simulink model "TwoBitMUX"  (R2017b)
settings: Solver=VariableStepAuto  StartTime=0.0  StopTime=10.0  RelTol=1e-3
libraries: hdlsllib x21
settings Model: Creator=Ray  LastModifiedBy=Ray

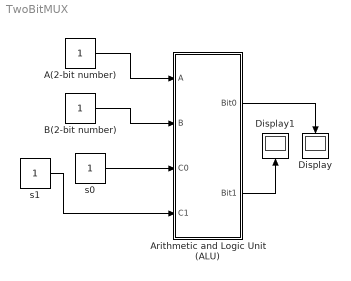
== system TwoBitMUX ==
  A(2-bit number) : Constant  OutDataTypeStr=uint8  SampleTime=1
  Arithmetic and Logic Unit (ALU) : Subsystem  TreatAsAtomicUnit=on
  B(2-bit number) : Constant  OutDataTypeStr=uint8  SampleTime=1
  Display : Display
  Display1 : Display
  s0 : Constant  OutDataTypeStr=boolean  SampleTime=1
  s1 : Constant  OutDataTypeStr=boolean  SampleTime=1
  wires:
  Arithmetic and Logic Unit (ALU)/1(Bit0) -> Display/1
  A(2-bit number)/1 -> Arithmetic and Logic Unit (ALU)/1(A)
  B(2-bit number)/1 -> Arithmetic and Logic Unit (ALU)/2(B)
  s0/1 -> Arithmetic and Logic Unit (ALU)/3(C0)
  s1/1 -> Arithmetic and Logic Unit (ALU)/4(C1)
  Arithmetic and Logic Unit (ALU)/2(Bit1) -> Display1/1

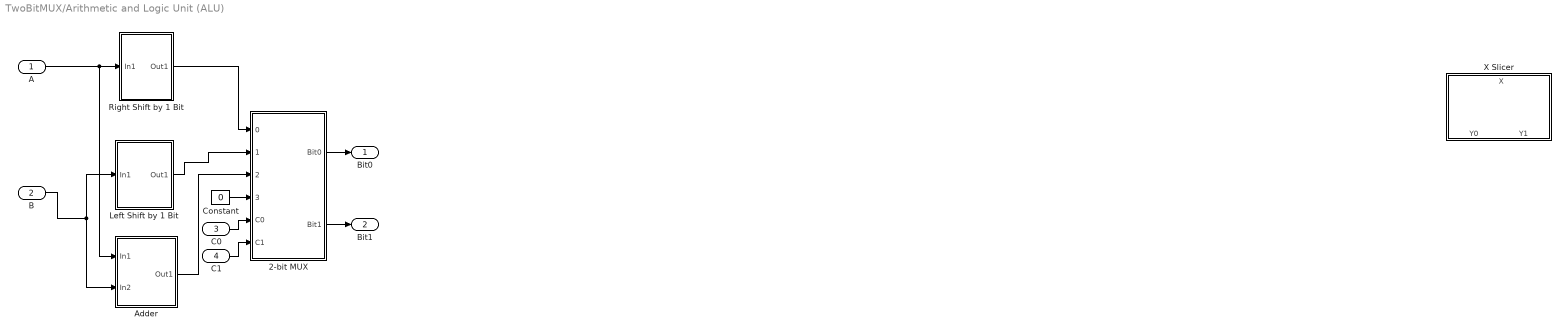
== system TwoBitMUX/Arithmetic and Logic Unit (ALU) ==
  A : Inport  OutDataTypeStr=uint8  SampleTime=1
  B : Inport  Port=2  OutDataTypeStr=uint8  SampleTime=1
  C0 : Inport  Port=3  OutDataTypeStr=boolean  SampleTime=1
  C1 : Inport  Port=4  OutDataTypeStr=boolean  SampleTime=1
  2-bit MUX : Subsystem
  Adder : Subsystem
  Constant : Constant  Value=0  OutDataTypeStr=uint8  SampleTime=1
  Left Shift by 1 Bit : Subsystem
  Right Shift by 1 Bit : Subsystem
  X Slicer : Subsystem
  Bit0 : Outport
  Bit1 : Outport  Port=2
  wires:
  Adder/1(Out1) -> 2-bit MUX/3(2)
  B/1 -> Adder/2(In2), Left Shift by 1 Bit/1(In1)
  A/1 -> Right Shift by 1 Bit/1(In1), Adder/1(In1)
  C0/1 -> 2-bit MUX/5(C0)
  C1/1 -> 2-bit MUX/6(C1)
  Constant/1 -> 2-bit MUX/4(3)
  2-bit MUX/1(Bit0) -> Bit0/1
  2-bit MUX/2(Bit1) -> Bit1/1
  Left Shift by 1 Bit/1(Out1) -> 2-bit MUX/2(1)
  Right Shift by 1 Bit/1(Out1) -> 2-bit MUX/1(0)

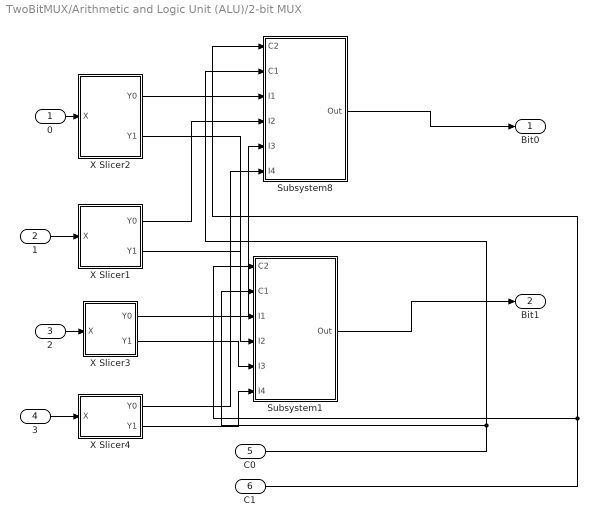
== system TwoBitMUX/Arithmetic and Logic Unit (ALU)/2-bit MUX ==
  0 : Inport  OutDataTypeStr=uint8  SampleTime=1
  1 : Inport  Port=2  OutDataTypeStr=uint8  SampleTime=1
  2 : Inport  Port=3  OutDataTypeStr=uint8  SampleTime=1
  3 : Inport  Port=4  OutDataTypeStr=uint8  SampleTime=1
  C0 : Inport  Port=5  OutDataTypeStr=boolean  SampleTime=1
  C1 : Inport  Port=6  OutDataTypeStr=boolean  SampleTime=1
  Subsystem1 : Subsystem
  Subsystem8 : Subsystem
  X Slicer1 : Subsystem
  X Slicer2 : Subsystem
  X Slicer3 : Subsystem
  X Slicer4 : Subsystem
  Bit0 : Outport  OutDataTypeStr=boolean  SampleTime=1
  Bit1 : Outport  Port=2  OutDataTypeStr=boolean  SampleTime=1
  wires:
  1/1 -> X Slicer1/1(X)
  X Slicer3/2(Y1) -> Subsystem1/5(I3)
  X Slicer1/1(Y0) -> Subsystem8/4(I2)
  X Slicer1/2(Y1) -> Subsystem1/4(I2)
  C1/1 -> Subsystem8/1(C2), Subsystem1/1(C2)
  X Slicer2/2(Y1) -> Subsystem1/3(I1)
  C0/1 -> Subsystem8/2(C1), Subsystem1/2(C1)
  X Slicer4/1(Y0) -> Subsystem8/6(I4)
  0/1 -> X Slicer2/1(X)
  X Slicer3/1(Y0) -> Subsystem8/5(I3)
  X Slicer4/2(Y1) -> Subsystem1/6(I4)
  X Slicer2/1(Y0) -> Subsystem8/3(I1)
  2/1 -> X Slicer3/1(X)
  3/1 -> X Slicer4/1(X)
  Subsystem8/1(Out) -> Bit0/1
  Subsystem1/1(Out) -> Bit1/1

== system TwoBitMUX/Arithmetic and Logic Unit (ALU)/Adder ==
  In1 : Inport
  In2 : Inport  Port=2
  8-bit Adder : Subsystem
  Bit Concat : Subsystem
  X Slicer : Subsystem
  X Slicer1 : Subsystem
  Out1 : Outport
  wires:
  Bit Concat/1(Out1) -> Out1/1
  In1/1 -> X Slicer/1(X)
  In2/1 -> X Slicer1/1(X)
  8-bit Adder/8(Out8) -> Bit Concat/1(In1)
  8-bit Adder/7(Out7) -> Bit Concat/2(In2)
  8-bit Adder/6(Out6) -> Bit Concat/3(In3)
  8-bit Adder/5(Out5) -> Bit Concat/4(In4)
  8-bit Adder/4(Out4) -> Bit Concat/5(In5)
  8-bit Adder/3(Out3) -> Bit Concat/6(In6)
  8-bit Adder/2(Out2) -> Bit Concat/7(In7)
  8-bit Adder/1(Out1) -> Bit Concat/8(In8)
  X Slicer/1(Y0) -> 8-bit Adder/1(A1)
  X Slicer/2(Y1) -> 8-bit Adder/3(A2)
  X Slicer1/1(Y0) -> 8-bit Adder/2(B1)
  X Slicer1/2(Y1) -> 8-bit Adder/10(B2)

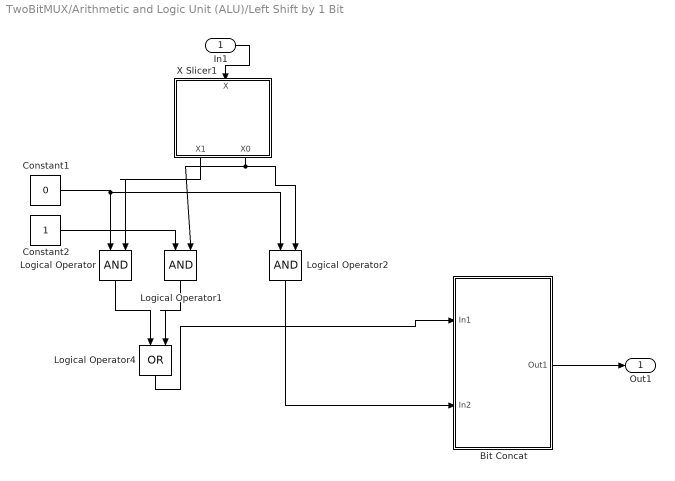
== system TwoBitMUX/Arithmetic and Logic Unit (ALU)/Left Shift by 1 Bit ==
  In1 : Inport
  Bit Concat : Subsystem
  Constant1 : Constant  Value=0  OutDataTypeStr=boolean  SampleTime=1
  Constant2 : Constant  OutDataTypeStr=boolean  SampleTime=1
  Logical Operator : Logic  IconShape=distinctive  AllPortsSameDT=off  OutDataTypeStr=boolean
  Logical Operator1 : Logic  IconShape=distinctive  AllPortsSameDT=off  OutDataTypeStr=boolean
  Logical Operator2 : Logic  IconShape=distinctive  AllPortsSameDT=off  OutDataTypeStr=boolean
  Logical Operator4 : Logic  Operator=OR  IconShape=distinctive  AllPortsSameDT=off  OutDataTypeStr=boolean
  X Slicer1 : Subsystem
  Out1 : Outport
  wires:
  Logical Operator4/1 -> Bit Concat/1(In1)
  X Slicer1/1(X1) -> Logical Operator/2
  Logical Operator2/1 -> Bit Concat/2(In2)
  Constant1/1 -> Logical Operator2/1, Logical Operator/1
  Logical Operator1/1 -> Logical Operator4/2
  X Slicer1/2(X0) -> Logical Operator2/2, Logical Operator1/2
  In1/1 -> X Slicer1/1(X)
  Constant2/1 -> Logical Operator1/1
  Logical Operator/1 -> Logical Operator4/1
  Bit Concat/1(Out1) -> Out1/1

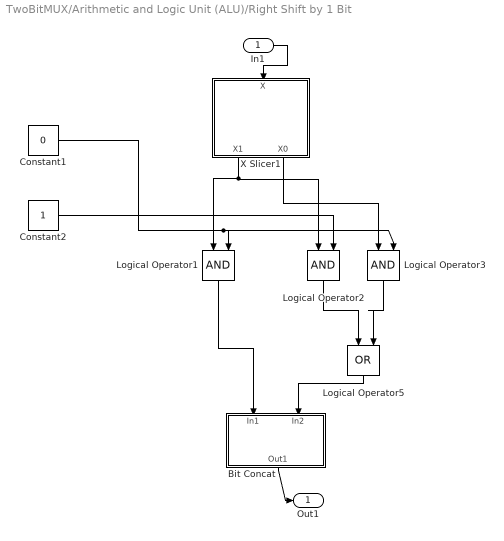
== system TwoBitMUX/Arithmetic and Logic Unit (ALU)/Right Shift by 1 Bit ==
  In1 : Inport
  Bit Concat : Subsystem
  Constant1 : Constant  Value=0  OutDataTypeStr=boolean  SampleTime=1
  Constant2 : Constant  OutDataTypeStr=boolean  SampleTime=1
  Logical Operator1 : Logic  IconShape=distinctive  AllPortsSameDT=off  OutDataTypeStr=boolean
  Logical Operator2 : Logic  IconShape=distinctive  AllPortsSameDT=off  OutDataTypeStr=boolean
  Logical Operator3 : Logic  IconShape=distinctive  AllPortsSameDT=off  OutDataTypeStr=boolean
  Logical Operator5 : Logic  Operator=OR  IconShape=distinctive  AllPortsSameDT=off  OutDataTypeStr=boolean
  X Slicer1 : Subsystem
  Out1 : Outport
  wires:
  In1/1 -> X Slicer1/1(X)
  Logical Operator5/1 -> Bit Concat/2(In2)
  Bit Concat/1(Out1) -> Out1/1
  X Slicer1/2(X0) -> Logical Operator3/1
  X Slicer1/1(X1) -> Logical Operator1/1, Logical Operator2/1
  Constant1/1 -> Logical Operator1/2, Logical Operator3/2
  Constant2/1 -> Logical Operator2/2
  Logical Operator1/1 -> Bit Concat/1(In1)
  Logical Operator3/1 -> Logical Operator5/2
  Logical Operator2/1 -> Logical Operator5/1

== system TwoBitMUX/Arithmetic and Logic Unit (ALU)/X Slicer ==
  X : Inport  OutDataTypeStr=uint8  SampleTime=1
  Bit Slice6 : hdlsllib/Logic and Bit Operations/Bit Slice  lidx=1  ridx=1
  Bit Slice7 : hdlsllib/Logic and Bit Operations/Bit Slice  lidx=0  ridx=0
  Data Type Conversion6 : DataTypeConversion  OutDataTypeStr=boolean
  Data Type Conversion7 : DataTypeConversion  OutDataTypeStr=boolean
  Y0 : Outport
  Y1 : Outport  Port=2
  wires:
  X/1 -> Bit Slice6/1, Bit Slice7/1
  Data Type Conversion6/1 -> Y1/1
  Bit Slice6/1 -> Data Type Conversion6/1
  Data Type Conversion7/1 -> Y0/1
  Bit Slice7/1 -> Data Type Conversion7/1

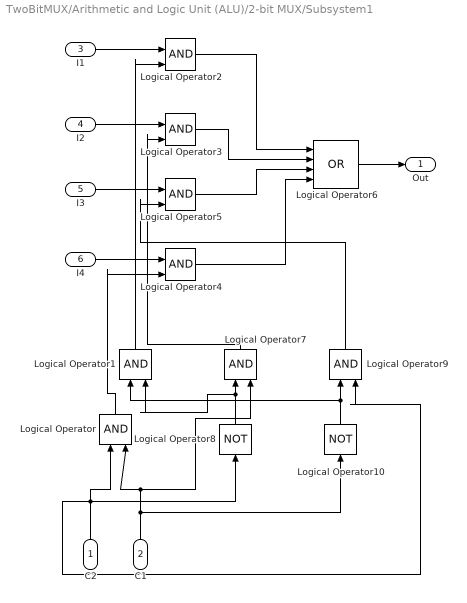
== system TwoBitMUX/Arithmetic and Logic Unit (ALU)/2-bit MUX/Subsystem1 ==
  C2 : Inport
  C1 : Inport  Port=2
  I1 : Inport  Port=3
  I2 : Inport  Port=4
  I3 : Inport  Port=5
  I4 : Inport  Port=6
  Logical Operator{,1..5,7,9} (8 alike) : Logic  IconShape=distinctive  AllPortsSameDT=off  OutDataTypeStr=boolean
  Logical Operator10 : Logic  Operator=NOT  IconShape=distinctive  AllPortsSameDT=off  OutDataTypeStr=boolean
  Logical Operator6 : Logic  Operator=OR  Inputs=4  IconShape=distinctive  AllPortsSameDT=off  OutDataTypeStr=boolean
  Logical Operator8 : Logic  Operator=NOT  IconShape=distinctive  AllPortsSameDT=off  OutDataTypeStr=boolean
  Out : Outport
  wires:
  I1/1 -> Logical Operator2/1
  I3/1 -> Logical Operator5/1
  Logical Operator4/1 -> Logical Operator6/4
  Logical Operator3/1 -> Logical Operator6/2
  C1/1 -> Logical Operator10/1, Logical Operator/2, Logical Operator7/2
  C2/1 -> Logical Operator9/2, Logical Operator/1, Logical Operator8/1
  Logical Operator10/1 -> Logical Operator1/1, Logical Operator9/1
  Logical Operator/1 -> Logical Operator4/2
  Logical Operator7/1 -> Logical Operator3/2
  I2/1 -> Logical Operator3/1
  Logical Operator2/1 -> Logical Operator6/1
  Logical Operator9/1 -> Logical Operator5/2
  I4/1 -> Logical Operator4/1
  Logical Operator5/1 -> Logical Operator6/3
  Logical Operator6/1 -> Out/1
  Logical Operator8/1 -> Logical Operator1/2, Logical Operator7/1
  Logical Operator1/1 -> Logical Operator2/2

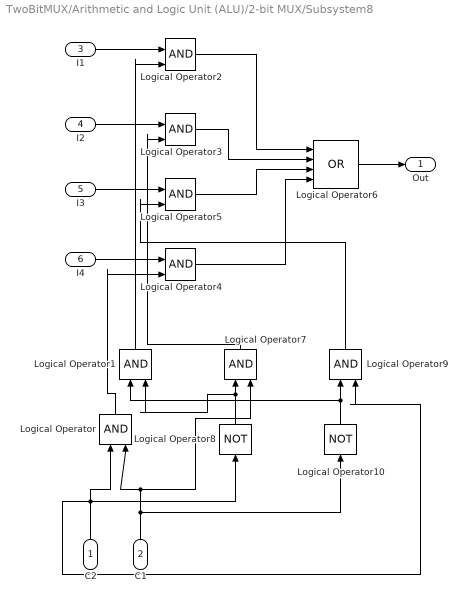
== system TwoBitMUX/Arithmetic and Logic Unit (ALU)/2-bit MUX/Subsystem8 ==
  C2 : Inport
  C1 : Inport  Port=2
  I1 : Inport  Port=3
  I2 : Inport  Port=4
  I3 : Inport  Port=5
  I4 : Inport  Port=6
  Logical Operator{,1..5,7,9} (8 alike) : Logic  IconShape=distinctive  AllPortsSameDT=off  OutDataTypeStr=boolean
  Logical Operator10 : Logic  Operator=NOT  IconShape=distinctive  AllPortsSameDT=off  OutDataTypeStr=boolean
  Logical Operator6 : Logic  Operator=OR  Inputs=4  IconShape=distinctive  AllPortsSameDT=off  OutDataTypeStr=boolean
  Logical Operator8 : Logic  Operator=NOT  IconShape=distinctive  AllPortsSameDT=off  OutDataTypeStr=boolean
  Out : Outport
  wires:
  I1/1 -> Logical Operator2/1
  I3/1 -> Logical Operator5/1
  Logical Operator4/1 -> Logical Operator6/4
  Logical Operator3/1 -> Logical Operator6/2
  C1/1 -> Logical Operator10/1, Logical Operator/2, Logical Operator7/2
  C2/1 -> Logical Operator9/2, Logical Operator/1, Logical Operator8/1
  Logical Operator10/1 -> Logical Operator1/1, Logical Operator9/1
  Logical Operator/1 -> Logical Operator4/2
  Logical Operator7/1 -> Logical Operator3/2
  I2/1 -> Logical Operator3/1
  Logical Operator2/1 -> Logical Operator6/1
  Logical Operator9/1 -> Logical Operator5/2
  I4/1 -> Logical Operator4/1
  Logical Operator5/1 -> Logical Operator6/3
  Logical Operator6/1 -> Out/1
  Logical Operator8/1 -> Logical Operator1/2, Logical Operator7/1
  Logical Operator1/1 -> Logical Operator2/2

== system TwoBitMUX/Arithmetic and Logic Unit (ALU)/2-bit MUX/X Slicer1 ==
  X : Inport  OutDataTypeStr=uint8  SampleTime=1
  Bit Slice6 : hdlsllib/Logic and Bit Operations/Bit Slice  lidx=1  ridx=1
  Bit Slice7 : hdlsllib/Logic and Bit Operations/Bit Slice  lidx=0  ridx=0
  Data Type Conversion6 : DataTypeConversion  OutDataTypeStr=boolean
  Data Type Conversion7 : DataTypeConversion  OutDataTypeStr=boolean
  Y0 : Outport  OutDataTypeStr=boolean  SampleTime=1
  Y1 : Outport  Port=2  OutDataTypeStr=boolean  SampleTime=1
  wires:
  X/1 -> Bit Slice6/1, Bit Slice7/1
  Data Type Conversion6/1 -> Y1/1
  Bit Slice6/1 -> Data Type Conversion6/1
  Data Type Conversion7/1 -> Y0/1
  Bit Slice7/1 -> Data Type Conversion7/1

== system TwoBitMUX/Arithmetic and Logic Unit (ALU)/2-bit MUX/X Slicer2 ==
  X : Inport  OutDataTypeStr=uint8  SampleTime=1
  Bit Slice6 : hdlsllib/Logic and Bit Operations/Bit Slice  lidx=1  ridx=1
  Bit Slice7 : hdlsllib/Logic and Bit Operations/Bit Slice  lidx=0  ridx=0
  Data Type Conversion6 : DataTypeConversion  OutDataTypeStr=boolean
  Data Type Conversion7 : DataTypeConversion  OutDataTypeStr=boolean
  Y0 : Outport  OutDataTypeStr=boolean  SampleTime=1
  Y1 : Outport  Port=2  OutDataTypeStr=boolean  SampleTime=1
  wires:
  X/1 -> Bit Slice6/1, Bit Slice7/1
  Data Type Conversion6/1 -> Y1/1
  Bit Slice6/1 -> Data Type Conversion6/1
  Data Type Conversion7/1 -> Y0/1
  Bit Slice7/1 -> Data Type Conversion7/1

== system TwoBitMUX/Arithmetic and Logic Unit (ALU)/2-bit MUX/X Slicer3 ==
  X : Inport  OutDataTypeStr=uint8  SampleTime=1
  Bit Slice6 : hdlsllib/Logic and Bit Operations/Bit Slice  lidx=1  ridx=1
  Bit Slice7 : hdlsllib/Logic and Bit Operations/Bit Slice  lidx=0  ridx=0
  Data Type Conversion6 : DataTypeConversion  OutDataTypeStr=boolean
  Data Type Conversion7 : DataTypeConversion  OutDataTypeStr=boolean
  Y0 : Outport  OutDataTypeStr=boolean  SampleTime=1
  Y1 : Outport  Port=2  OutDataTypeStr=boolean  SampleTime=1
  wires:
  X/1 -> Bit Slice6/1, Bit Slice7/1
  Data Type Conversion6/1 -> Y1/1
  Bit Slice6/1 -> Data Type Conversion6/1
  Data Type Conversion7/1 -> Y0/1
  Bit Slice7/1 -> Data Type Conversion7/1

== system TwoBitMUX/Arithmetic and Logic Unit (ALU)/2-bit MUX/X Slicer4 ==
  X : Inport  OutDataTypeStr=uint8  SampleTime=1
  Bit Slice6 : hdlsllib/Logic and Bit Operations/Bit Slice  lidx=1  ridx=1
  Bit Slice7 : hdlsllib/Logic and Bit Operations/Bit Slice  lidx=0  ridx=0
  Data Type Conversion6 : DataTypeConversion  OutDataTypeStr=boolean
  Data Type Conversion7 : DataTypeConversion  OutDataTypeStr=boolean
  Y0 : Outport  OutDataTypeStr=boolean  SampleTime=1
  Y1 : Outport  Port=2  OutDataTypeStr=boolean  SampleTime=1
  wires:
  X/1 -> Bit Slice6/1, Bit Slice7/1
  Data Type Conversion6/1 -> Y1/1
  Bit Slice6/1 -> Data Type Conversion6/1
  Data Type Conversion7/1 -> Y0/1
  Bit Slice7/1 -> Data Type Conversion7/1

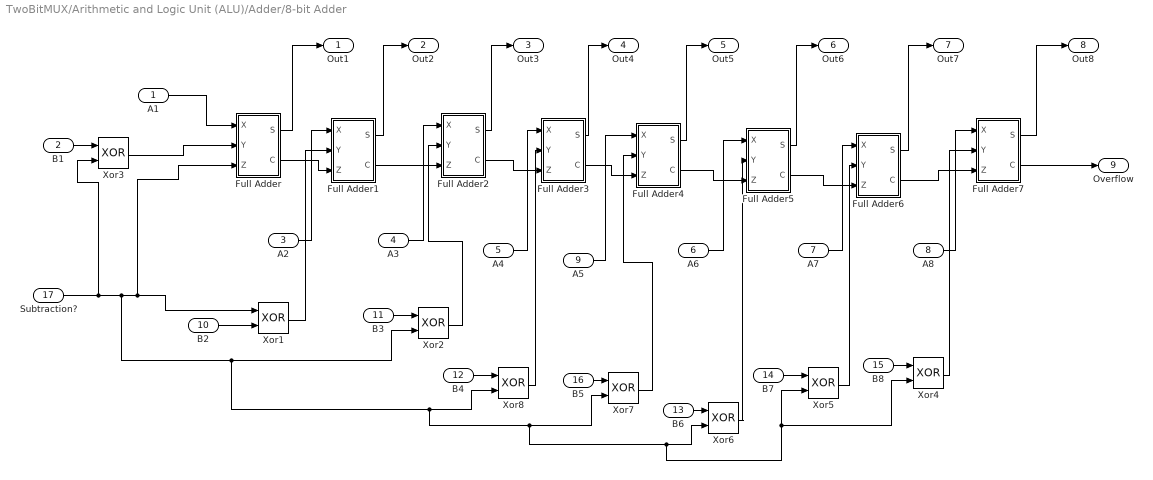
== system TwoBitMUX/Arithmetic and Logic Unit (ALU)/Adder/8-bit Adder ==
  A1 : Inport
  B1 : Inport  Port=2
  A2 : Inport  Port=3
  A3 : Inport  Port=4
  A4 : Inport  Port=5
  A6 : Inport  Port=6
  A7 : Inport  Port=7
  A8 : Inport  Port=8
  A5 : Inport  Port=9
  B2 : Inport  Port=10
  B3 : Inport  Port=11
  B4 : Inport  Port=12
  B6 : Inport  Port=13
  B7 : Inport  Port=14
  B8 : Inport  Port=15
  B5 : Inport  Port=16
  Subtraction? : Inport  Port=17  OutDataTypeStr=boolean
  Full Adder : Subsystem
  Full Adder1 : Subsystem
  Full Adder2 : Subsystem
  Full Adder3 : Subsystem
  Full Adder4 : Subsystem
  Full Adder5 : Subsystem
  Full Adder6 : Subsystem
  Full Adder7 : Subsystem
  Xor{1..8} (8 alike) : Logic  Operator=XOR  AllPortsSameDT=off  OutDataTypeStr=boolean
  Out1 : Outport  OutDataTypeStr=boolean
  Out2 : Outport  Port=2  OutDataTypeStr=boolean
  Out3 : Outport  Port=3  OutDataTypeStr=boolean
  Out4 : Outport  Port=4  OutDataTypeStr=boolean
  Out5 : Outport  Port=5  OutDataTypeStr=boolean
  Out6 : Outport  Port=6  OutDataTypeStr=boolean
  Out7 : Outport  Port=7  OutDataTypeStr=boolean
  Out8 : Outport  Port=8  OutDataTypeStr=boolean
  Overflow : Outport  Port=9  OutDataTypeStr=boolean
  wires:
  Full Adder7/2(C) -> Overflow/1
  Full Adder5/2(C) -> Full Adder6/3(Z)
  Full Adder7/1(S) -> Out8/1
  Full Adder4/2(C) -> Full Adder5/3(Z)
  Full Adder/2(C) -> Full Adder1/3(Z)
  Full Adder6/2(C) -> Full Adder7/3(Z)
  Full Adder6/1(S) -> Out7/1
  Full Adder2/2(C) -> Full Adder3/3(Z)
  Full Adder4/1(S) -> Out5/1
  A2/1 -> Full Adder1/1(X)
  A5/1 -> Full Adder4/1(X)
  Full Adder1/1(S) -> Out2/1
  A7/1 -> Full Adder6/1(X)
  Full Adder5/1(S) -> Out6/1
  A1/1 -> Full Adder/1(X)
  A8/1 -> Full Adder7/1(X)
  A6/1 -> Full Adder5/1(X)
  A4/1 -> Full Adder3/1(X)
  Full Adder3/1(S) -> Out4/1
  Full Adder/1(S) -> Out1/1
  Full Adder1/2(C) -> Full Adder2/3(Z)
  A3/1 -> Full Adder2/1(X)
  Full Adder3/2(C) -> Full Adder4/3(Z)
  Full Adder2/1(S) -> Out3/1
  B2/1 -> Xor1/2
  Subtraction?/1 -> Xor3/2, Xor4/2, Xor5/2, Xor6/2, Xor7/2, Xor8/2, Xor2/2, Full Adder/3(Z), Xor1/1
  Xor1/1 -> Full Adder1/2(Y)
  Xor2/1 -> Full Adder2/2(Y)
  B3/1 -> Xor2/1
  B4/1 -> Xor8/1
  Xor8/1 -> Full Adder3/2(Y)
  B5/1 -> Xor7/1
  Xor7/1 -> Full Adder4/2(Y)
  B6/1 -> Xor6/1
  Xor6/1 -> Full Adder5/2(Y)
  B7/1 -> Xor5/1
  Xor5/1 -> Full Adder6/2(Y)
  Xor4/1 -> Full Adder7/2(Y)
  B8/1 -> Xor4/1
  Xor3/1 -> Full Adder/2(Y)
  B1/1 -> Xor3/1

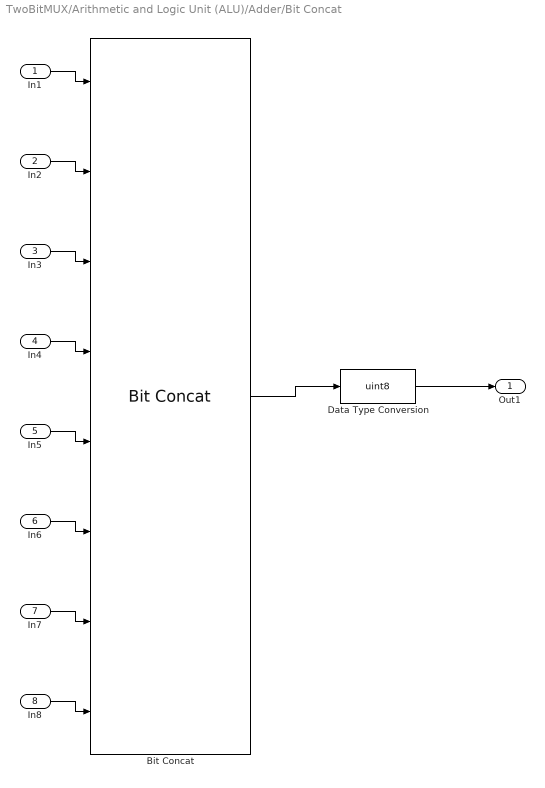
== system TwoBitMUX/Arithmetic and Logic Unit (ALU)/Adder/Bit Concat ==
  In1 : Inport
  In2 : Inport  Port=2
  In3 : Inport  Port=3
  In4 : Inport  Port=4
  In5 : Inport  Port=5
  In6 : Inport  Port=6
  In7 : Inport  Port=7
  In8 : Inport  Port=8
  Bit Concat : hdlsllib/Logic and Bit Operations/Bit Concat  numInputs=8
      settings: SourceProductName=HDL Coder  SourceProductBaseCode=HD
  Data Type Conversion : DataTypeConversion  OutDataTypeStr=uint8
  Out1 : Outport
  wires:
  Data Type Conversion/1 -> Out1/1
  In1/1 -> Bit Concat/1
  In4/1 -> Bit Concat/4
  In2/1 -> Bit Concat/2
  In3/1 -> Bit Concat/3
  In5/1 -> Bit Concat/5
  In6/1 -> Bit Concat/6
  In7/1 -> Bit Concat/7
  In8/1 -> Bit Concat/8
  Bit Concat/1 -> Data Type Conversion/1

== system TwoBitMUX/Arithmetic and Logic Unit (ALU)/Adder/X Slicer ==
  X : Inport  OutDataTypeStr=uint8  SampleTime=1
  Bit Slice6 : hdlsllib/Logic and Bit Operations/Bit Slice  lidx=1  ridx=1
  Bit Slice7 : hdlsllib/Logic and Bit Operations/Bit Slice  lidx=0  ridx=0
  Data Type Conversion6 : DataTypeConversion  OutDataTypeStr=boolean
  Data Type Conversion7 : DataTypeConversion  OutDataTypeStr=boolean
  Y0 : Outport
  Y1 : Outport  Port=2
  wires:
  X/1 -> Bit Slice6/1, Bit Slice7/1
  Data Type Conversion6/1 -> Y1/1
  Bit Slice6/1 -> Data Type Conversion6/1
  Data Type Conversion7/1 -> Y0/1
  Bit Slice7/1 -> Data Type Conversion7/1

== system TwoBitMUX/Arithmetic and Logic Unit (ALU)/Adder/X Slicer1 ==
  X : Inport  OutDataTypeStr=uint8  SampleTime=1
  Bit Slice6 : hdlsllib/Logic and Bit Operations/Bit Slice  lidx=1  ridx=1
  Bit Slice7 : hdlsllib/Logic and Bit Operations/Bit Slice  lidx=0  ridx=0
  Data Type Conversion6 : DataTypeConversion  OutDataTypeStr=boolean
  Data Type Conversion7 : DataTypeConversion  OutDataTypeStr=boolean
  Y0 : Outport
  Y1 : Outport  Port=2
  wires:
  X/1 -> Bit Slice6/1, Bit Slice7/1
  Data Type Conversion6/1 -> Y1/1
  Bit Slice6/1 -> Data Type Conversion6/1
  Data Type Conversion7/1 -> Y0/1
  Bit Slice7/1 -> Data Type Conversion7/1

== system TwoBitMUX/Arithmetic and Logic Unit (ALU)/Left Shift by 1 Bit/Bit Concat ==
  In1 : Inport
  In2 : Inport  Port=2
  Bit Concat : hdlsllib/Logic and Bit Operations/Bit Concat  numInputs=2
      settings: SourceProductName=HDL Coder  SourceProductBaseCode=HD
  Data Type Conversion : DataTypeConversion  OutDataTypeStr=uint8
  Out1 : Outport
  wires:
  Data Type Conversion/1 -> Out1/1
  Bit Concat/1 -> Data Type Conversion/1
  In2/1 -> Bit Concat/2
  In1/1 -> Bit Concat/1

== system TwoBitMUX/Arithmetic and Logic Unit (ALU)/Left Shift by 1 Bit/X Slicer1 ==
  X : Inport  OutDataTypeStr=uint8  SampleTime=1
  Bit Slice6 : hdlsllib/Logic and Bit Operations/Bit Slice  lidx=1  ridx=1
  Bit Slice7 : hdlsllib/Logic and Bit Operations/Bit Slice  lidx=0  ridx=0
  Data Type Conversion6 : DataTypeConversion  OutDataTypeStr=boolean
  Data Type Conversion7 : DataTypeConversion  OutDataTypeStr=boolean
  X1 : Outport
  X0 : Outport  Port=2
  wires:
  X/1 -> Bit Slice6/1, Bit Slice7/1
  Data Type Conversion6/1 -> X1/1
  Bit Slice6/1 -> Data Type Conversion6/1
  Data Type Conversion7/1 -> X0/1
  Bit Slice7/1 -> Data Type Conversion7/1

== system TwoBitMUX/Arithmetic and Logic Unit (ALU)/Right Shift by 1 Bit/Bit Concat ==
  In1 : Inport
  In2 : Inport  Port=2
  Bit Concat : hdlsllib/Logic and Bit Operations/Bit Concat  numInputs=2
      settings: SourceProductName=HDL Coder  SourceProductBaseCode=HD
  Data Type Conversion : DataTypeConversion  OutDataTypeStr=uint8
  Out1 : Outport
  wires:
  Data Type Conversion/1 -> Out1/1
  Bit Concat/1 -> Data Type Conversion/1
  In2/1 -> Bit Concat/2
  In1/1 -> Bit Concat/1

== system TwoBitMUX/Arithmetic and Logic Unit (ALU)/Right Shift by 1 Bit/X Slicer1 ==
  X : Inport  OutDataTypeStr=uint8  SampleTime=1
  Bit Slice6 : hdlsllib/Logic and Bit Operations/Bit Slice  lidx=1  ridx=1
  Bit Slice7 : hdlsllib/Logic and Bit Operations/Bit Slice  lidx=0  ridx=0
  Data Type Conversion6 : DataTypeConversion  OutDataTypeStr=boolean
  Data Type Conversion7 : DataTypeConversion  OutDataTypeStr=boolean
  X1 : Outport
  X0 : Outport  Port=2
  wires:
  X/1 -> Bit Slice6/1, Bit Slice7/1
  Data Type Conversion6/1 -> X1/1
  Bit Slice6/1 -> Data Type Conversion6/1
  Data Type Conversion7/1 -> X0/1
  Bit Slice7/1 -> Data Type Conversion7/1

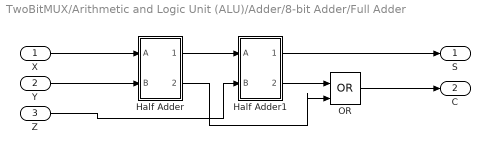
== system TwoBitMUX/Arithmetic and Logic Unit (ALU)/Adder/8-bit Adder/Full Adder ==
  X : Inport
  Y : Inport  Port=2
  Z : Inport  Port=3
  Half Adder : Subsystem
  Half Adder1 : Subsystem
  OR : Logic  Operator=OR  IconShape=distinctive  AllPortsSameDT=off  OutDataTypeStr=boolean
  S : Outport
  C : Outport  Port=2
  wires:
  Half Adder1/1(Sum) -> S/1
  Half Adder/1(Sum) -> Half Adder1/1(A)
  Half Adder/2(Carry) -> OR/2
  X/1 -> Half Adder/1(A)
  Z/1 -> Half Adder1/2(B)
  OR/1 -> C/1
  Y/1 -> Half Adder/2(B)
  Half Adder1/2(Carry) -> OR/1

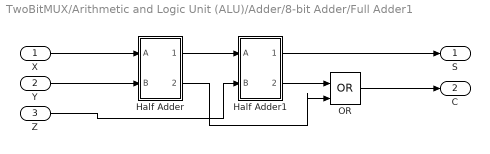
== system TwoBitMUX/Arithmetic and Logic Unit (ALU)/Adder/8-bit Adder/Full Adder1 ==
  X : Inport
  Y : Inport  Port=2
  Z : Inport  Port=3
  Half Adder : Subsystem
  Half Adder1 : Subsystem
  OR : Logic  Operator=OR  IconShape=distinctive  AllPortsSameDT=off  OutDataTypeStr=boolean
  S : Outport
  C : Outport  Port=2
  wires:
  Half Adder1/1(Sum) -> S/1
  Half Adder/1(Sum) -> Half Adder1/1(A)
  Half Adder/2(Carry) -> OR/2
  X/1 -> Half Adder/1(A)
  Z/1 -> Half Adder1/2(B)
  OR/1 -> C/1
  Y/1 -> Half Adder/2(B)
  Half Adder1/2(Carry) -> OR/1

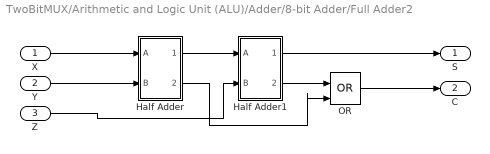
== system TwoBitMUX/Arithmetic and Logic Unit (ALU)/Adder/8-bit Adder/Full Adder2 ==
  X : Inport
  Y : Inport  Port=2
  Z : Inport  Port=3
  Half Adder : Subsystem
  Half Adder1 : Subsystem
  OR : Logic  Operator=OR  IconShape=distinctive  AllPortsSameDT=off  OutDataTypeStr=boolean
  S : Outport
  C : Outport  Port=2
  wires:
  Half Adder1/1(Sum) -> S/1
  Half Adder/1(Sum) -> Half Adder1/1(A)
  Half Adder/2(Carry) -> OR/2
  X/1 -> Half Adder/1(A)
  Z/1 -> Half Adder1/2(B)
  OR/1 -> C/1
  Y/1 -> Half Adder/2(B)
  Half Adder1/2(Carry) -> OR/1

== system TwoBitMUX/Arithmetic and Logic Unit (ALU)/Adder/8-bit Adder/Full Adder3 ==
  X : Inport
  Y : Inport  Port=2
  Z : Inport  Port=3
  Half Adder : Subsystem
  Half Adder1 : Subsystem
  OR : Logic  Operator=OR  IconShape=distinctive  AllPortsSameDT=off  OutDataTypeStr=boolean
  S : Outport
  C : Outport  Port=2
  wires:
  Half Adder1/1(Sum) -> S/1
  Half Adder/1(Sum) -> Half Adder1/1(A)
  Half Adder/2(Carry) -> OR/2
  X/1 -> Half Adder/1(A)
  Z/1 -> Half Adder1/2(B)
  OR/1 -> C/1
  Y/1 -> Half Adder/2(B)
  Half Adder1/2(Carry) -> OR/1

== system TwoBitMUX/Arithmetic and Logic Unit (ALU)/Adder/8-bit Adder/Full Adder4 ==
  X : Inport
  Y : Inport  Port=2
  Z : Inport  Port=3
  Half Adder : Subsystem
  Half Adder1 : Subsystem
  OR : Logic  Operator=OR  IconShape=distinctive  AllPortsSameDT=off  OutDataTypeStr=boolean
  S : Outport
  C : Outport  Port=2
  wires:
  Half Adder1/1(Sum) -> S/1
  Half Adder/1(Sum) -> Half Adder1/1(A)
  Half Adder/2(Carry) -> OR/2
  X/1 -> Half Adder/1(A)
  Z/1 -> Half Adder1/2(B)
  OR/1 -> C/1
  Y/1 -> Half Adder/2(B)
  Half Adder1/2(Carry) -> OR/1

== system TwoBitMUX/Arithmetic and Logic Unit (ALU)/Adder/8-bit Adder/Full Adder5 ==
  X : Inport
  Y : Inport  Port=2
  Z : Inport  Port=3
  Half Adder : Subsystem
  Half Adder1 : Subsystem
  OR : Logic  Operator=OR  IconShape=distinctive  AllPortsSameDT=off  OutDataTypeStr=boolean
  S : Outport
  C : Outport  Port=2
  wires:
  Half Adder1/1(Sum) -> S/1
  Half Adder/1(Sum) -> Half Adder1/1(A)
  Half Adder/2(Carry) -> OR/2
  X/1 -> Half Adder/1(A)
  Z/1 -> Half Adder1/2(B)
  OR/1 -> C/1
  Y/1 -> Half Adder/2(B)
  Half Adder1/2(Carry) -> OR/1

== system TwoBitMUX/Arithmetic and Logic Unit (ALU)/Adder/8-bit Adder/Full Adder6 ==
  X : Inport
  Y : Inport  Port=2
  Z : Inport  Port=3
  Half Adder : Subsystem
  Half Adder1 : Subsystem
  OR : Logic  Operator=OR  IconShape=distinctive  AllPortsSameDT=off  OutDataTypeStr=boolean
  S : Outport
  C : Outport  Port=2
  wires:
  Half Adder1/1(Sum) -> S/1
  Half Adder/1(Sum) -> Half Adder1/1(A)
  Half Adder/2(Carry) -> OR/2
  X/1 -> Half Adder/1(A)
  Z/1 -> Half Adder1/2(B)
  OR/1 -> C/1
  Y/1 -> Half Adder/2(B)
  Half Adder1/2(Carry) -> OR/1

== system TwoBitMUX/Arithmetic and Logic Unit (ALU)/Adder/8-bit Adder/Full Adder7 ==
  X : Inport
  Y : Inport  Port=2
  Z : Inport  Port=3
  Half Adder : Subsystem
  Half Adder1 : Subsystem
  OR : Logic  Operator=OR  IconShape=distinctive  AllPortsSameDT=off  OutDataTypeStr=boolean
  S : Outport
  C : Outport  Port=2
  wires:
  Half Adder1/1(Sum) -> S/1
  Half Adder/1(Sum) -> Half Adder1/1(A)
  Half Adder/2(Carry) -> OR/2
  X/1 -> Half Adder/1(A)
  Z/1 -> Half Adder1/2(B)
  OR/1 -> C/1
  Y/1 -> Half Adder/2(B)
  Half Adder1/2(Carry) -> OR/1

== system TwoBitMUX/Arithmetic and Logic Unit (ALU)/Adder/8-bit Adder/Full Adder/Half Adder ==
  A : Inport
  B : Inport  Port=2
  AND : Logic  IconShape=distinctive  AllPortsSameDT=off  OutDataTypeStr=boolean
  XOR : Logic  Operator=XOR  IconShape=distinctive  AllPortsSameDT=off  OutDataTypeStr=boolean
  Sum : Outport
  Carry : Outport  Port=2
  wires:
  AND/1 -> Carry/1
  XOR/1 -> Sum/1
  B/1 -> XOR/2, AND/2
  A/1 -> AND/1, XOR/1

== system TwoBitMUX/Arithmetic and Logic Unit (ALU)/Adder/8-bit Adder/Full Adder/Half Adder1 ==
  A : Inport
  B : Inport  Port=2
  AND : Logic  IconShape=distinctive  AllPortsSameDT=off  OutDataTypeStr=boolean
  XOR : Logic  Operator=XOR  IconShape=distinctive  AllPortsSameDT=off  OutDataTypeStr=boolean
  Sum : Outport
  Carry : Outport  Port=2
  wires:
  AND/1 -> Carry/1
  XOR/1 -> Sum/1
  B/1 -> XOR/2, AND/2
  A/1 -> AND/1, XOR/1

== system TwoBitMUX/Arithmetic and Logic Unit (ALU)/Adder/8-bit Adder/Full Adder1/Half Adder ==
  A : Inport
  B : Inport  Port=2
  AND : Logic  IconShape=distinctive  AllPortsSameDT=off  OutDataTypeStr=boolean
  XOR : Logic  Operator=XOR  IconShape=distinctive  AllPortsSameDT=off  OutDataTypeStr=boolean
  Sum : Outport
  Carry : Outport  Port=2
  wires:
  AND/1 -> Carry/1
  XOR/1 -> Sum/1
  B/1 -> XOR/2, AND/2
  A/1 -> AND/1, XOR/1

== system TwoBitMUX/Arithmetic and Logic Unit (ALU)/Adder/8-bit Adder/Full Adder1/Half Adder1 ==
  A : Inport
  B : Inport  Port=2
  AND : Logic  IconShape=distinctive  AllPortsSameDT=off  OutDataTypeStr=boolean
  XOR : Logic  Operator=XOR  IconShape=distinctive  AllPortsSameDT=off  OutDataTypeStr=boolean
  Sum : Outport
  Carry : Outport  Port=2
  wires:
  AND/1 -> Carry/1
  XOR/1 -> Sum/1
  B/1 -> XOR/2, AND/2
  A/1 -> AND/1, XOR/1

== system TwoBitMUX/Arithmetic and Logic Unit (ALU)/Adder/8-bit Adder/Full Adder2/Half Adder ==
  A : Inport
  B : Inport  Port=2
  AND : Logic  IconShape=distinctive  AllPortsSameDT=off  OutDataTypeStr=boolean
  XOR : Logic  Operator=XOR  IconShape=distinctive  AllPortsSameDT=off  OutDataTypeStr=boolean
  Sum : Outport
  Carry : Outport  Port=2
  wires:
  AND/1 -> Carry/1
  XOR/1 -> Sum/1
  B/1 -> XOR/2, AND/2
  A/1 -> AND/1, XOR/1

== system TwoBitMUX/Arithmetic and Logic Unit (ALU)/Adder/8-bit Adder/Full Adder2/Half Adder1 ==
  A : Inport
  B : Inport  Port=2
  AND : Logic  IconShape=distinctive  AllPortsSameDT=off  OutDataTypeStr=boolean
  XOR : Logic  Operator=XOR  IconShape=distinctive  AllPortsSameDT=off  OutDataTypeStr=boolean
  Sum : Outport
  Carry : Outport  Port=2
  wires:
  AND/1 -> Carry/1
  XOR/1 -> Sum/1
  B/1 -> XOR/2, AND/2
  A/1 -> AND/1, XOR/1

== system TwoBitMUX/Arithmetic and Logic Unit (ALU)/Adder/8-bit Adder/Full Adder3/Half Adder ==
  A : Inport
  B : Inport  Port=2
  AND : Logic  IconShape=distinctive  AllPortsSameDT=off  OutDataTypeStr=boolean
  XOR : Logic  Operator=XOR  IconShape=distinctive  AllPortsSameDT=off  OutDataTypeStr=boolean
  Sum : Outport
  Carry : Outport  Port=2
  wires:
  AND/1 -> Carry/1
  XOR/1 -> Sum/1
  B/1 -> XOR/2, AND/2
  A/1 -> AND/1, XOR/1

== system TwoBitMUX/Arithmetic and Logic Unit (ALU)/Adder/8-bit Adder/Full Adder3/Half Adder1 ==
  A : Inport
  B : Inport  Port=2
  AND : Logic  IconShape=distinctive  AllPortsSameDT=off  OutDataTypeStr=boolean
  XOR : Logic  Operator=XOR  IconShape=distinctive  AllPortsSameDT=off  OutDataTypeStr=boolean
  Sum : Outport
  Carry : Outport  Port=2
  wires:
  AND/1 -> Carry/1
  XOR/1 -> Sum/1
  B/1 -> XOR/2, AND/2
  A/1 -> AND/1, XOR/1

== system TwoBitMUX/Arithmetic and Logic Unit (ALU)/Adder/8-bit Adder/Full Adder4/Half Adder ==
  A : Inport
  B : Inport  Port=2
  AND : Logic  IconShape=distinctive  AllPortsSameDT=off  OutDataTypeStr=boolean
  XOR : Logic  Operator=XOR  IconShape=distinctive  AllPortsSameDT=off  OutDataTypeStr=boolean
  Sum : Outport
  Carry : Outport  Port=2
  wires:
  AND/1 -> Carry/1
  XOR/1 -> Sum/1
  B/1 -> XOR/2, AND/2
  A/1 -> AND/1, XOR/1

== system TwoBitMUX/Arithmetic and Logic Unit (ALU)/Adder/8-bit Adder/Full Adder4/Half Adder1 ==
  A : Inport
  B : Inport  Port=2
  AND : Logic  IconShape=distinctive  AllPortsSameDT=off  OutDataTypeStr=boolean
  XOR : Logic  Operator=XOR  IconShape=distinctive  AllPortsSameDT=off  OutDataTypeStr=boolean
  Sum : Outport
  Carry : Outport  Port=2
  wires:
  AND/1 -> Carry/1
  XOR/1 -> Sum/1
  B/1 -> XOR/2, AND/2
  A/1 -> AND/1, XOR/1

== system TwoBitMUX/Arithmetic and Logic Unit (ALU)/Adder/8-bit Adder/Full Adder5/Half Adder ==
  A : Inport
  B : Inport  Port=2
  AND : Logic  IconShape=distinctive  AllPortsSameDT=off  OutDataTypeStr=boolean
  XOR : Logic  Operator=XOR  IconShape=distinctive  AllPortsSameDT=off  OutDataTypeStr=boolean
  Sum : Outport
  Carry : Outport  Port=2
  wires:
  AND/1 -> Carry/1
  XOR/1 -> Sum/1
  B/1 -> XOR/2, AND/2
  A/1 -> AND/1, XOR/1

== system TwoBitMUX/Arithmetic and Logic Unit (ALU)/Adder/8-bit Adder/Full Adder5/Half Adder1 ==
  A : Inport
  B : Inport  Port=2
  AND : Logic  IconShape=distinctive  AllPortsSameDT=off  OutDataTypeStr=boolean
  XOR : Logic  Operator=XOR  IconShape=distinctive  AllPortsSameDT=off  OutDataTypeStr=boolean
  Sum : Outport
  Carry : Outport  Port=2
  wires:
  AND/1 -> Carry/1
  XOR/1 -> Sum/1
  B/1 -> XOR/2, AND/2
  A/1 -> AND/1, XOR/1

== system TwoBitMUX/Arithmetic and Logic Unit (ALU)/Adder/8-bit Adder/Full Adder6/Half Adder ==
  A : Inport
  B : Inport  Port=2
  AND : Logic  IconShape=distinctive  AllPortsSameDT=off  OutDataTypeStr=boolean
  XOR : Logic  Operator=XOR  IconShape=distinctive  AllPortsSameDT=off  OutDataTypeStr=boolean
  Sum : Outport
  Carry : Outport  Port=2
  wires:
  AND/1 -> Carry/1
  XOR/1 -> Sum/1
  B/1 -> XOR/2, AND/2
  A/1 -> AND/1, XOR/1

== system TwoBitMUX/Arithmetic and Logic Unit (ALU)/Adder/8-bit Adder/Full Adder6/Half Adder1 ==
  A : Inport
  B : Inport  Port=2
  AND : Logic  IconShape=distinctive  AllPortsSameDT=off  OutDataTypeStr=boolean
  XOR : Logic  Operator=XOR  IconShape=distinctive  AllPortsSameDT=off  OutDataTypeStr=boolean
  Sum : Outport
  Carry : Outport  Port=2
  wires:
  AND/1 -> Carry/1
  XOR/1 -> Sum/1
  B/1 -> XOR/2, AND/2
  A/1 -> AND/1, XOR/1

== system TwoBitMUX/Arithmetic and Logic Unit (ALU)/Adder/8-bit Adder/Full Adder7/Half Adder ==
  A : Inport
  B : Inport  Port=2
  AND : Logic  IconShape=distinctive  AllPortsSameDT=off  OutDataTypeStr=boolean
  XOR : Logic  Operator=XOR  IconShape=distinctive  AllPortsSameDT=off  OutDataTypeStr=boolean
  Sum : Outport
  Carry : Outport  Port=2
  wires:
  AND/1 -> Carry/1
  XOR/1 -> Sum/1
  B/1 -> XOR/2, AND/2
  A/1 -> AND/1, XOR/1

== system TwoBitMUX/Arithmetic and Logic Unit (ALU)/Adder/8-bit Adder/Full Adder7/Half Adder1 ==
  A : Inport
  B : Inport  Port=2
  AND : Logic  IconShape=distinctive  AllPortsSameDT=off  OutDataTypeStr=boolean
  XOR : Logic  Operator=XOR  IconShape=distinctive  AllPortsSameDT=off  OutDataTypeStr=boolean
  Sum : Outport
  Carry : Outport  Port=2
  wires:
  AND/1 -> Carry/1
  XOR/1 -> Sum/1
  B/1 -> XOR/2, AND/2
  A/1 -> AND/1, XOR/1
